simulink model "lap2"  (R2022b)
settings: Solver=VariableStepAuto  StartTime=0.0  StopTime=20  RelTol=1e-3
settings Model: Creator=yasso  LastModifiedBy=yasso

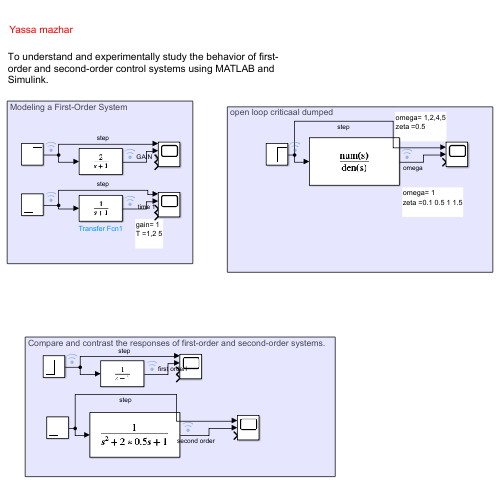
[thumbnail: Simulink's stored preview of the top-level diagram]
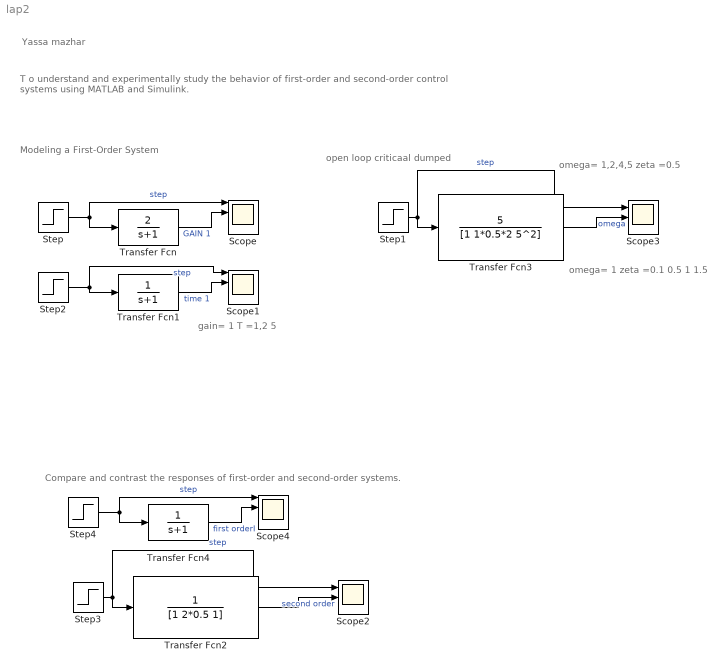
== system lap2 ==
  note: Compare and contrast the responses of first-order and second-order systems.
  note: omega= 1,2,4,5
      | zeta =0.5
  note: Modeling a First-Order System
  note: Yassa mazhar
  note: T o understand and experimentally study the behavior of first-order and second-order control systems using MATLAB and Simulink.
  note: open loop criticaal dumped
  note: gain= 1
      | T =1,2 5
  note: omega= 1
      | zeta =0.1 0.5 1 1.5
  Scope : Scope  NumInputPorts=4
  Scope1 : Scope  NumInputPorts=4
  Scope2 : Scope  NumInputPorts=3
  Scope3 : Scope  NumInputPorts=3
  Scope4 : Scope  NumInputPorts=4
  Step{,1..4} (5 alike) : Step  SampleTime=0
  Transfer Fcn : TransferFcn  Numerator=2  Denominator=[1 1]
  Transfer Fcn1 : TransferFcn  Numerator=1  Denominator=[1 1]
  Transfer Fcn2 : TransferFcn  Numerator=1  Denominator=[1 2*0.5 1]
  Transfer Fcn3 : TransferFcn  Numerator=5  Denominator=[1 1*0.5*2 5^2]
  Transfer Fcn4 : TransferFcn  Numerator=1  Denominator=[1 1]
  wires:
  Transfer Fcn/1 -> Scope/2  "GAIN 1"
  Step/1 -> Transfer Fcn/1, Scope/1  "step"
  Transfer Fcn3/1 -> Scope3/2  "omega"
  Step1/1 -> Transfer Fcn3/1, Scope3/1  "step"
  Step2/1 -> Scope1/1, Transfer Fcn1/1  "step"
  Transfer Fcn1/1 -> Scope1/2  "time 1"
  Step3/1 -> Scope2/1, Transfer Fcn2/1  "step"
  Transfer Fcn2/1 -> Scope2/2  "second order"
  Step4/1 -> Scope4/1, Transfer Fcn4/1  "step"
  Transfer Fcn4/1 -> Scope4/2  "first orderI"
